simulink model "example"  (R2023b)
settings: Solver=FixedStepDiscrete  StartTime=0.0  StopTime=10.0  RelTol=1e-3
model workspace (MAT data in the model file):
  firstWarning = 1
  originalScenarioChecksum = 'E8518274013465E46D92F4550C671EFC'
undefined symbols (not defined in the file or in its folder): driving
libraries: drivingscenarioandsensors x16
(part 1 of 5)
settings Model: Creator=nc1yellow  LastModifiedBy=nc1yellow

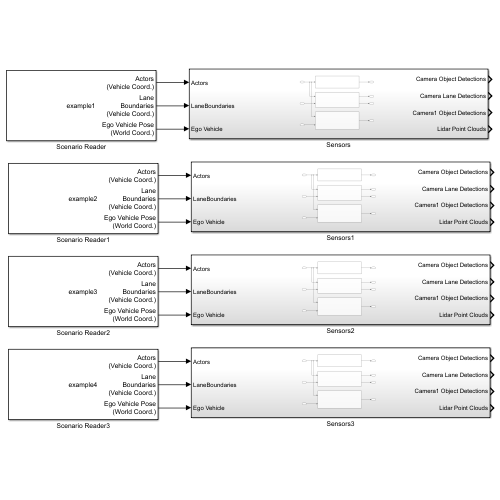
[thumbnail: Simulink's stored preview of the top-level diagram]
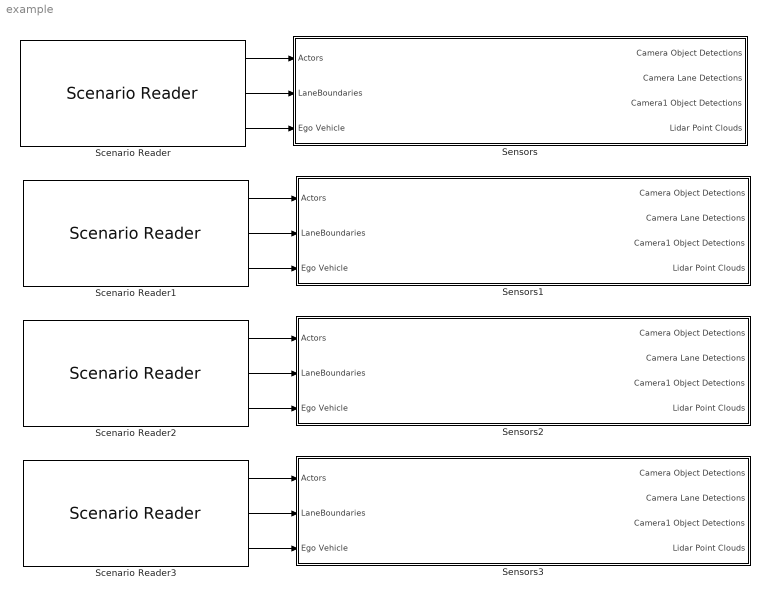
== system example ==
  Scenario Reader : drivingscenarioandsensors/Scenario Reader  ScenarioSource=From file  ScenarioFileName=C:\Users\nc1yellow\Documents\MATLAB\Examples\R2023b\autonomous_control\AdaptiveCruiseControlWithSensorFusionExample\example\example1.mat  ScenarioVariableName=scenario  OutputCoordinateSystem=Vehicle coordinates  EgoVehicleSource=Scenario  EgoVehicleActorID=1  OrientVehiclesOnRoad=off  OutputEgoVehiclePose=on  OutputEgoVehicleState=off  SampleTime=0.1  LaneBoundaryOutput=Ego vehicle lane boundaries  LaneBoundaryDistance=linspace(-100, 100, 101)  LaneBoundaryLocation=Center of lane markings  BusNameSource=Auto  BusName=BusActors  BusNumActorsSource=Scenario  BusNumActors=100  BusName2Source=Auto  BusName2=BusLaneBoundaries  BusNumLaneBoundariesSource=Scenario  BusNumLaneBoundaries=10  BusName3Source=Auto  BusName3=BusEgoActor  BusName4Source=Auto  BusName4=BusEgoState  ShowCoordinateLabels=on  SimulateUsing=Interpreted execution
  Scenario Reader1 : drivingscenarioandsensors/Scenario Reader  ScenarioSource=From file  ScenarioFileName=C:\Users\nc1yellow\Documents\MATLAB\Examples\R2023b\autonomous_control\AdaptiveCruiseControlWithSensorFusionExample\example\example2.mat  ScenarioVariableName=scenario  OutputCoordinateSystem=Vehicle coordinates  EgoVehicleSource=Scenario  EgoVehicleActorID=1  OrientVehiclesOnRoad=off  OutputEgoVehiclePose=on  OutputEgoVehicleState=off  SampleTime=0.1  LaneBoundaryOutput=Ego vehicle lane boundaries  LaneBoundaryDistance=linspace(-100, 100, 101)  LaneBoundaryLocation=Center of lane markings  BusNameSource=Auto  BusName=BusActors  BusNumActorsSource=Scenario  BusNumActors=100  BusName2Source=Auto  BusName2=BusLaneBoundaries  BusNumLaneBoundariesSource=Scenario  BusNumLaneBoundaries=10  BusName3Source=Auto  BusName3=BusEgoActor  BusName4Source=Auto  BusName4=BusEgoState  ShowCoordinateLabels=on  SimulateUsing=Interpreted execution
  Scenario Reader2 : drivingscenarioandsensors/Scenario Reader  ScenarioSource=From file  ScenarioFileName=C:\Users\nc1yellow\Documents\MATLAB\Examples\R2023b\autonomous_control\AdaptiveCruiseControlWithSensorFusionExample\example\example3.mat  ScenarioVariableName=scenario  OutputCoordinateSystem=Vehicle coordinates  EgoVehicleSource=Scenario  EgoVehicleActorID=1  OrientVehiclesOnRoad=off  OutputEgoVehiclePose=on  OutputEgoVehicleState=off  SampleTime=0.1  LaneBoundaryOutput=Ego vehicle lane boundaries  LaneBoundaryDistance=linspace(-100, 100, 101)  LaneBoundaryLocation=Center of lane markings  BusNameSource=Auto  BusName=BusActors  BusNumActorsSource=Scenario  BusNumActors=100  BusName2Source=Auto  BusName2=BusLaneBoundaries  BusNumLaneBoundariesSource=Scenario  BusNumLaneBoundaries=10  BusName3Source=Auto  BusName3=BusEgoActor  BusName4Source=Auto  BusName4=BusEgoState  ShowCoordinateLabels=on  SimulateUsing=Interpreted execution
  Scenario Reader3 : drivingscenarioandsensors/Scenario Reader  ScenarioSource=From file  ScenarioFileName=C:\Users\nc1yellow\Documents\MATLAB\Examples\R2023b\autonomous_control\AdaptiveCruiseControlWithSensorFusionExample\example\example4.mat  ScenarioVariableName=scenario  OutputCoordinateSystem=Vehicle coordinates  EgoVehicleSource=Scenario  EgoVehicleActorID=1  OrientVehiclesOnRoad=off  OutputEgoVehiclePose=on  OutputEgoVehicleState=off  SampleTime=0.1  LaneBoundaryOutput=Ego vehicle lane boundaries  LaneBoundaryDistance=linspace(-100, 100, 101)  LaneBoundaryLocation=Center of lane markings  BusNameSource=Auto  BusName=BusActors  BusNumActorsSource=Scenario  BusNumActors=100  BusName2Source=Auto  BusName2=BusLaneBoundaries  BusNumLaneBoundariesSource=Scenario  BusNumLaneBoundaries=10  BusName3Source=Auto  BusName3=BusEgoActor  BusName4Source=Auto  BusName4=BusEgoState  ShowCoordinateLabels=on  SimulateUsing=Interpreted execution
  Sensors : Subsystem
  Sensors1 : Subsystem
  Sensors2 : Subsystem
  Sensors3 : Subsystem
  wires:
  Scenario Reader/1 -> Sensors/1(Actors)
  Scenario Reader/2 -> Sensors/2(LaneBoundaries)
  Scenario Reader/3 -> Sensors/3(Ego Vehicle)
  Scenario Reader1/3 -> Sensors1/3(Ego Vehicle)
  Scenario Reader1/2 -> Sensors1/2(LaneBoundaries)
  Scenario Reader1/1 -> Sensors1/1(Actors)
  Scenario Reader2/1 -> Sensors2/1(Actors)
  Scenario Reader2/2 -> Sensors2/2(LaneBoundaries)
  Scenario Reader2/3 -> Sensors2/3(Ego Vehicle)
  Scenario Reader3/1 -> Sensors3/1(Actors)
  Scenario Reader3/3 -> Sensors3/3(Ego Vehicle)
  Scenario Reader3/2 -> Sensors3/2(LaneBoundaries)
